simulink model "Model_without_motor"  (R2024b)
settings: Solver=VariableStepAuto  StartTime=0.0  StopTime=5  RelTol=1e-3
values from neighbouring files (symbols this model uses):
  g = 9.81    [main.m]
  L = 0.5    [main.m]
  m0 = 2    [main.m]
  m1 = 0.5    [main.m]
settings Model: Creator=Anfisa Konycheva  LastModifiedBy=Anfisa Konycheva

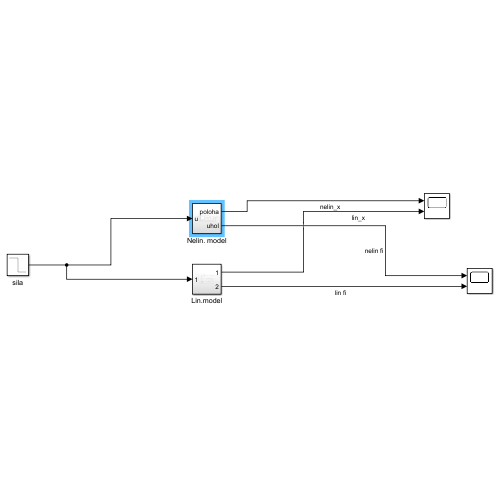
[thumbnail: Simulink's stored preview of the top-level diagram]
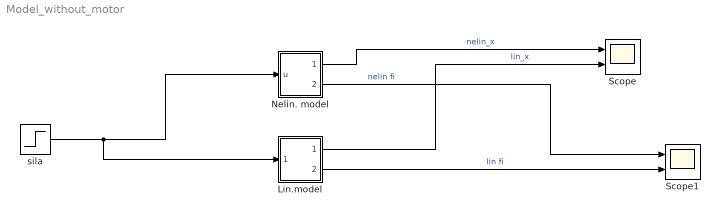
== system Model_without_motor ==
  Lin.model : Subsystem
  Nelin. model : Subsystem
  Scope : Scope  NumInputPorts=2
  Scope1 : Scope  NumInputPorts=2
  sila : Step  Before=1  After=0  SampleTime=0
  wires:
  sila/1 -> Lin.model/1(In1), Nelin. model/1(u)
  Nelin. model/1(poloha) -> Scope/1  "nelin_x"
  Nelin. model/2(uhol) -> Scope1/1  "nelin fi"
  Lin.model/1(Out1) -> Scope/2  "lin_x"
  Lin.model/2(Out2) -> Scope1/2  "lin fi"

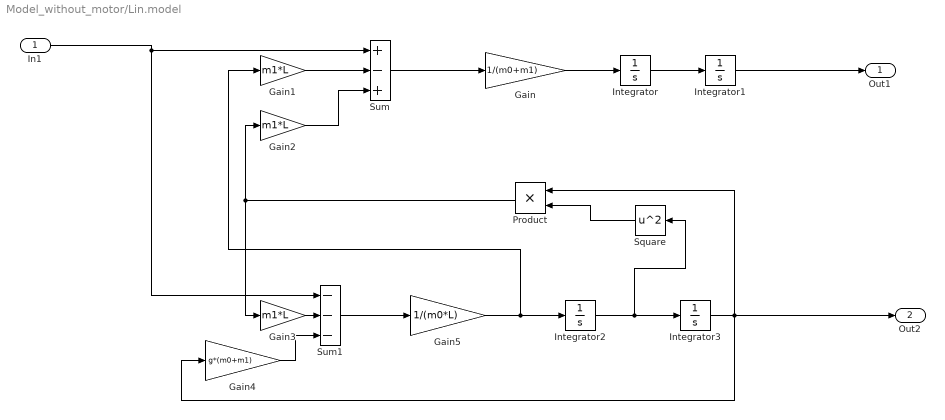
== system Model_without_motor/Lin.model ==
  In1 : Inport
  Gain : Gain  Gain=1/(m0+m1)
  Gain1 : Gain  Gain=m1*L
  Gain2 : Gain  Gain=m1*L
  Gain3 : Gain  Gain=m1*L
  Gain4 : Gain  Gain=g*(m0+m1)
  Gain5 : Gain  Gain=1/(m0*L)
  Integrator{,1..3} (4 alike) : Integrator
  Product : Product
  Square : Math  Operator=square
  Sum : Sum  Inputs=+-+
  Sum1 : Sum  Inputs=---
  Out1 : Outport
  Out2 : Outport  Port=2
  wires:
  Square/1 -> Product/2
  In1/1 -> Sum1/1, Sum/1
  Gain4/1 -> Sum1/3
  Integrator3/1 -> Out2/1, Product/1, Gain4/1
  Gain3/1 -> Sum1/2
  Integrator/1 -> Integrator1/1
  Product/1 -> Gain3/1, Gain2/1
  Gain1/1 -> Sum/2
  Integrator1/1 -> Out1/1
  Gain2/1 -> Sum/3
  Gain/1 -> Integrator/1
  Sum/1 -> Gain/1
  Gain5/1 -> Gain1/1, Integrator2/1
  Integrator2/1 -> Square/1, Integrator3/1
  Sum1/1 -> Gain5/1

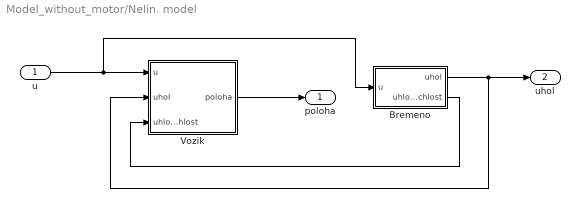
== system Model_without_motor/Nelin. model ==
  u : Inport
  Bremeno : Subsystem
  Vozik : Subsystem
  poloha : Outport
  uhol : Outport  Port=2
  wires:
  u/1 -> Bremeno/1(u), Vozik/1(u)
  Vozik/1(poloha) -> poloha/1
  Bremeno/1(uhol) -> uhol/1, Vozik/2(uhol)
  Bremeno/2(uhlova rychlost) -> Vozik/3(uhlova rychlost)

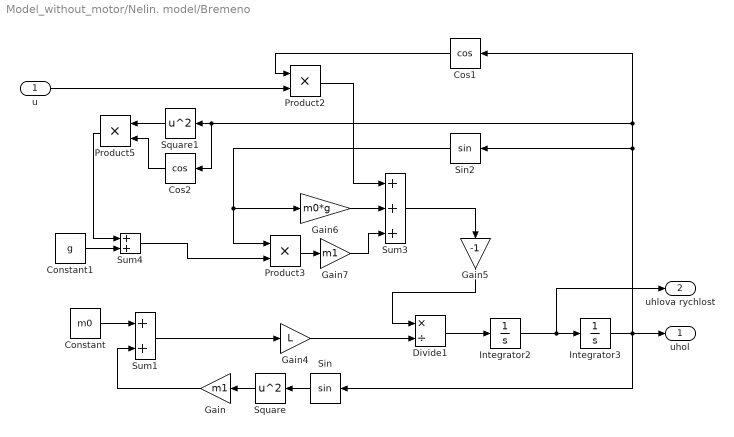
== system Model_without_motor/Nelin. model/Bremeno ==
  u : Inport
  Constant : Constant  Value=m0
  Constant1 : Constant  Value=g
  Cos1 : Trigonometry  Operator=cos
  Cos2 : Trigonometry  Operator=cos
  Divide1 : Product  Inputs=*/
  Gain : Gain  Gain=m1
  Gain4 : Gain  Gain=L
  Gain5 : Gain  Gain=-1
  Gain6 : Gain  Gain=m0*g
  Gain7 : Gain  Gain=m1
  Integrator2 : Integrator
  Integrator3 : Integrator
  Product2 : Product
  Product3 : Product
  Product5 : Product
  Sin : Trigonometry
  Sin2 : Trigonometry
  Square : Math  Operator=square
  Square1 : Math  Operator=square
  Sum1 : Sum
  Sum3 : Sum  Inputs=+++
  Sum4 : Sum
  uhol : Outport
  uhlova rychlost : Outport  Port=2
  wires:
  Product5/1 -> Sum4/1
  Gain6/1 -> Sum3/2
  Sum3/1 -> Gain5/1
  Constant1/1 -> Sum4/2
  Sum1/1 -> Gain4/1
  Gain7/1 -> Sum3/3
  Gain5/1 -> Divide1/1
  Product3/1 -> Gain7/1
  Cos2/1 -> Product5/2
  Product2/1 -> Sum3/1
  Sum4/1 -> Product3/2
  Divide1/1 -> Integrator2/1
  Sin2/1 -> Gain6/1, Product3/1
  Gain4/1 -> Divide1/2
  Integrator2/1 -> uhlova rychlost/1, Integrator3/1
  Cos1/1 -> Product2/1
  u/1 -> Product2/2
  Square1/1 -> Product5/1
  Square/1 -> Gain/1
  Constant/1 -> Sum1/1
  Sin/1 -> Square/1
  Gain/1 -> Sum1/2
  Integrator3/1 -> Sin/1, uhol/1, Cos1/1, Cos2/1, Square1/1, Sin2/1

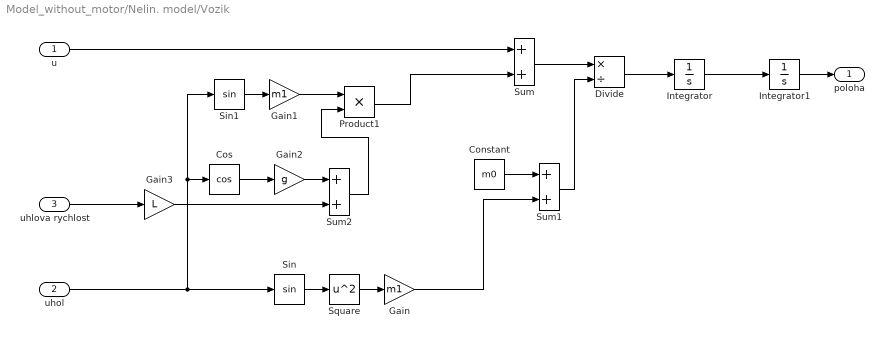
== system Model_without_motor/Nelin. model/Vozik ==
  u : Inport
  uhol : Inport  Port=2
  uhlova rychlost : Inport  Port=3
  Constant : Constant  Value=m0
  Cos : Trigonometry  Operator=cos
  Divide : Product  Inputs=*/
  Gain : Gain  Gain=m1
  Gain1 : Gain  Gain=m1
  Gain2 : Gain  Gain=g
  Gain3 : Gain  Gain=L
  Integrator : Integrator
  Integrator1 : Integrator
  Product1 : Product
  Sin : Trigonometry
  Sin1 : Trigonometry
  Square : Math  Operator=square
  Sum : Sum
  Sum1 : Sum
  Sum2 : Sum
  poloha : Outport
  wires:
  Product1/1 -> Sum/2
  Gain1/1 -> Product1/1
  Sin/1 -> Square/1
  Cos/1 -> Gain2/1
  uhol/1 -> Sin/1, Sin1/1, Cos/1
  Integrator/1 -> Integrator1/1
  Sum/1 -> Divide/1
  Divide/1 -> Integrator/1
  Sum1/1 -> Divide/2
  Sum2/1 -> Product1/2
  Gain2/1 -> Sum2/1
  Gain/1 -> Sum1/2
  Constant/1 -> Sum1/1
  Sin1/1 -> Gain1/1
  Gain3/1 -> Sum2/2
  Square/1 -> Gain/1
  Integrator1/1 -> poloha/1
  uhlova rychlost/1 -> Gain3/1
  u/1 -> Sum/1
